simulink model "simulation_composite"  (Simulink 6.6)
settings: Solver=ode45  StartTime=0.0  StopTime=10.0  RelTol=1e-3
values from neighbouring files (symbols this model uses):
  desired_states = [set_point.theta; set_point.omega]    [set_parameters.m]    (also in tablesat3.m = str2num(get(handles.set_points,'String')))
  measurement_noise = evalin('base','measurement_noise')    [tablesat3.m]
  PID = evalin('base','PID')    [tablesat3.m]
  process_noise = evalin('base','process_noise')    [tablesat3.m]
undefined symbols (not defined in the file or in its folder): flag, plant
settings Model: Creator=Cooch  LastModifiedBy=Administrator
settings DebuggingCC: AlgebraicLoopMsg=none  SolverPrmCheckMsg=none  UnconnectedInputMsg=none  UnconnectedOutputMsg=none  UnconnectedLineMsg=none

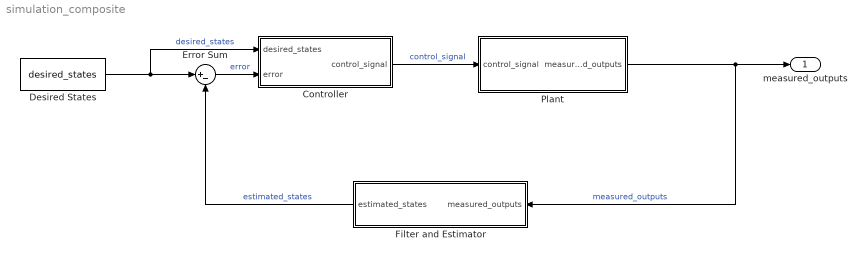
== system simulation_composite ==
  Controller : Subsystem
  Desired States : Constant  Value=desired_states
  Error Sum : Sum  Inputs=|+-
  Filter and Estimator : Subsystem  Orientation=left
  Plant : Subsystem
  measured_outputs : Outport
  wires:
  Desired States/1 -> Error Sum/1, Controller/1(desired_states)  "desired_states"
  Error Sum/1 -> Controller/2(error)  "error"
  Controller/1(control_signal) -> Plant/1(control_signal)  "control_signal"
  Filter and Estimator/1(estimated_states) -> Error Sum/2  "estimated_states"
  Plant/1(measured_outputs) -> Filter and Estimator/1(measured_outputs), measured_outputs/1  "measured_outputs"

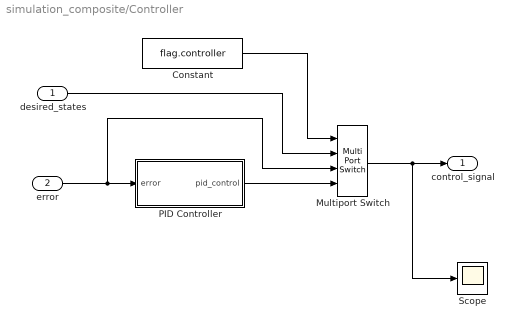
== system simulation_composite/Controller ==
  desired_states : Inport
  error : Inport  Port=2
  Constant : Constant  Value=flag.controller
  Multiport Switch : MultiPortSwitch  Inputs=3  zeroidx=on
  PID Controller : Subsystem
  Scope : Scope
  control_signal : Outport
  wires:
  error/1 -> PID Controller/1(error), Multiport Switch/3
  Multiport Switch/1 -> control_signal/1, Scope/1
  Constant/1 -> Multiport Switch/1
  PID Controller/1(pid_control) -> Multiport Switch/4
  desired_states/1 -> Multiport Switch/2

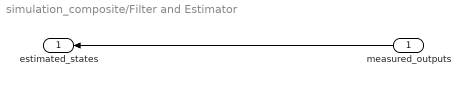
== system simulation_composite/Filter and Estimator ==
  measured_outputs : Inport  Orientation=left
  estimated_states : Outport  Orientation=left
  wires:
  measured_outputs/1 -> estimated_states/1

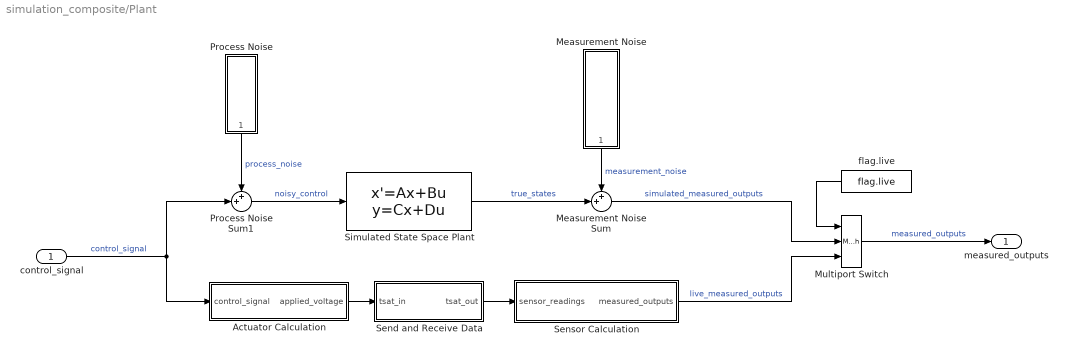
== system simulation_composite/Plant ==
  control_signal : Inport
  Actuator Calculation : Subsystem
  Measurement Noise : Subsystem  Orientation=down
  Measurement Noise Sum : Sum  Inputs=++|
  Multiport Switch : MultiPortSwitch  Inputs=2  zeroidx=on
  Process Noise : Subsystem  Orientation=down
  Process Noise Sum1 : Sum  Inputs=++|
  Send and Receive Data : Subsystem
  Sensor Calculation : Subsystem
  Simulated State Space Plant : StateSpace  A=plant.A  B=plant.B  C=plant.C  D=plant.D  X0=plant.ic
  flag.live : Constant  Orientation=left  Value=flag.live
  measured_outputs : Outport
  wires:
  Actuator Calculation/1(applied_voltage) -> Send and Receive Data/1(tsat_in)
  Send and Receive Data/1(tsat_out) -> Sensor Calculation/1(sensor_readings)
  Measurement Noise/1(measurement_noise) -> Measurement Noise Sum/1  "measurement_noise"
  Simulated State Space Plant/1 -> Measurement Noise Sum/2  "true_states"
  Multiport Switch/1 -> measured_outputs/1  "measured_outputs"
  flag.live/1 -> Multiport Switch/1
  Measurement Noise Sum/1 -> Multiport Switch/2  "simulated_measured_outputs"
  Sensor Calculation/1(measured_outputs) -> Multiport Switch/3  "live_measured_outputs"
  Process Noise/1(process_noise) -> Process Noise Sum1/1  "process_noise"
  Process Noise Sum1/1 -> Simulated State Space Plant/1  "noisy_control"
  control_signal/1 -> Process Noise Sum1/2, Actuator Calculation/1(control_signal)  "control_signal"

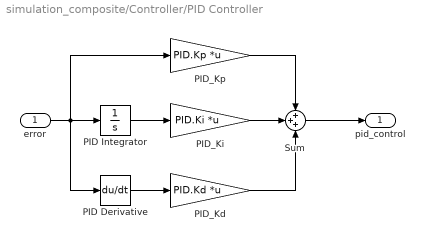
== system simulation_composite/Controller/PID Controller ==
  error : Inport
  PID Derivative : Derivative
  PID Integrator : Integrator
  PID_Kd : Gain  Gain=PID.Kd  Multiplication=Matrix(K*u)
  PID_Ki : Gain  Gain=PID.Ki  Multiplication=Matrix(K*u)
  PID_Kp : Gain  Gain=PID.Kp  Multiplication=Matrix(K*u)
  Sum : Sum  Inputs=+++
  pid_control : Outport
  wires:
  PID Integrator/1 -> PID_Ki/1
  PID Derivative/1 -> PID_Kd/1
  PID_Kp/1 -> Sum/1
  error/1 -> PID_Kp/1, PID Integrator/1, PID Derivative/1
  PID_Ki/1 -> Sum/2
  PID_Kd/1 -> Sum/3
  Sum/1 -> pid_control/1

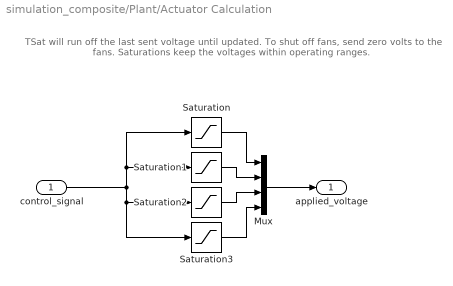
== system simulation_composite/Plant/Actuator Calculation ==
  note: TSat will run off the last sent voltage until updated.
      | To shut off fans, send zero volts to the fans.
      |
      | Saturations keep the voltages within operating ranges.
  control_signal : Inport
  Mux : Mux
  Saturation{,1..3} (4 alike) : Saturate  UpperLimit=12  LowerLimit=0
  applied_voltage : Outport
  wires:
  control_signal/1 -> Saturation/1, Saturation1/1, Saturation2/1, Saturation3/1
  Saturation/1 -> Mux/1
  Saturation1/1 -> Mux/2
  Saturation2/1 -> Mux/3
  Saturation3/1 -> Mux/4
  Mux/1 -> applied_voltage/1

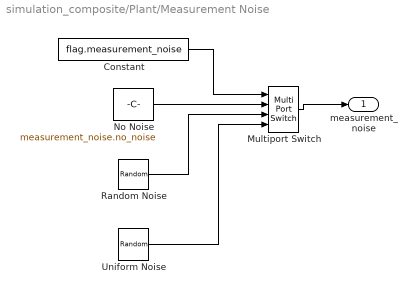
== system simulation_composite/Plant/Measurement Noise ==
  Constant : Constant  Value=flag.measurement_noise
  Multiport Switch : MultiPortSwitch  Inputs=3  zeroidx=on
  No Noise : Constant  Value=measurement_noise.no_noise
  Random Noise : RandomNumber  Mean=measurement_noise.random.mean  Variance=measurement_noise.random.variance  SampleTime=0
  Uniform Noise : UniformRandomNumber  Minimum=measurement_noise.uniform.min  Maximum=measurement_noise.uniform.max  SampleTime=0
  measurement_noise : Outport
  wires:
  Uniform Noise/1 -> Multiport Switch/4
  Constant/1 -> Multiport Switch/1
  No Noise/1 -> Multiport Switch/2
  Random Noise/1 -> Multiport Switch/3
  Multiport Switch/1 -> measurement_noise/1

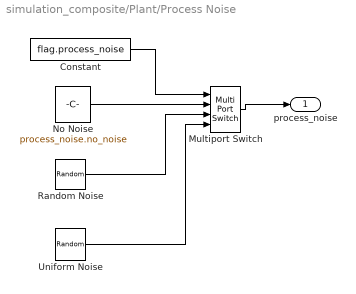
== system simulation_composite/Plant/Process Noise ==
  Constant : Constant  Value=flag.process_noise
  Multiport Switch : MultiPortSwitch  Inputs=3  zeroidx=on
  No Noise : Constant  Value=process_noise.no_noise
  Random Noise : RandomNumber  Mean=process_noise.random.mean  Variance=process_noise.random.variance  SampleTime=0
  Uniform Noise : UniformRandomNumber  Minimum=process_noise.uniform.min  Maximum=process_noise.uniform.max  SampleTime=0
  process_noise : Outport
  wires:
  Constant/1 -> Multiport Switch/1
  No Noise/1 -> Multiport Switch/2
  Random Noise/1 -> Multiport Switch/3
  Multiport Switch/1 -> process_noise/1
  Uniform Noise/1 -> Multiport Switch/4

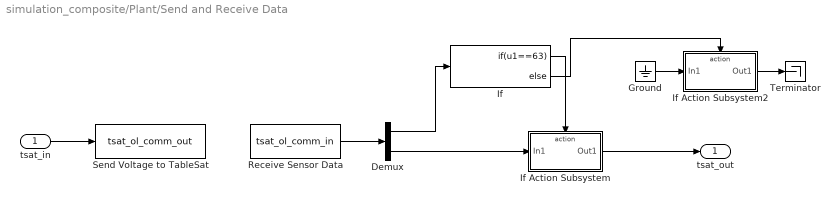
== system simulation_composite/Plant/Send and Receive Data ==
  tsat_in : Inport
  Demux : Demux  Outputs=[1;-1]
  Ground : Ground
  If : If  IfExpression=u1==63
  If Action Subsystem : Subsystem  TreatAsAtomicUnit=on
  If Action Subsystem2 : Subsystem  TreatAsAtomicUnit=on
  Receive Sensor Data : S-Function  FunctionName=tsat_ol_comm_in
  Send Voltage to TableSat : S-Function  FunctionName=tsat_ol_comm_out
  Terminator : Terminator
  tsat_out : Outport
  wires:
  tsat_in/1 -> Send Voltage to TableSat/1
  If/1 -> If Action Subsystem/Action
  If/2 -> If Action Subsystem2/Action
  Demux/1 -> If/1
  Receive Sensor Data/1 -> Demux/1
  If Action Subsystem2/1(Out1) -> Terminator/1
  Demux/2 -> If Action Subsystem/1(In1)
  Ground/1 -> If Action Subsystem2/1(In1)
  If Action Subsystem/1(Out1) -> tsat_out/1

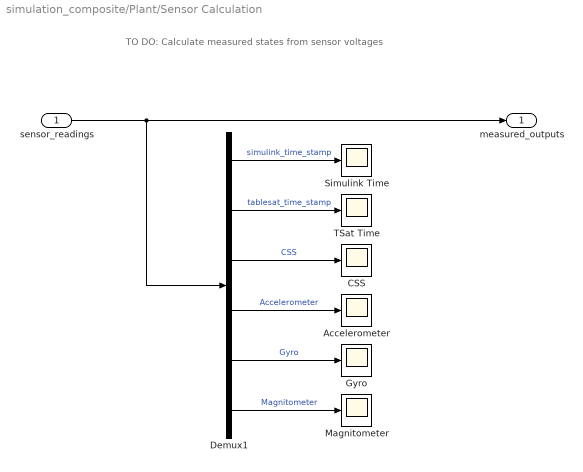
== system simulation_composite/Plant/Sensor Calculation ==
  note: TO DO: Calculate measured states from sensor voltages
  sensor_readings : Inport
  Accelerometer : Scope
      settings: YMin=2.5  YMax=4.25  SaveName=ScopeData4
  CSS : Scope
      settings: SaveName=ScopeData3
  Demux1 : Demux  Outputs=[1;1;6;4;1;3]
  Gyro : Scope
      settings: SaveName=ScopeData5
  Magnitometer : Scope
      settings: SaveName=ScopeData6
  Simulink Time : Scope
      settings: TimeRange=10  YMin=0  YMax=10
  TSat Time : Scope
      settings: SaveName=ScopeData2
  measured_outputs : Outport
  wires:
  Demux1/1 -> Simulink Time/1  "simulink_time_stamp"
  Demux1/2 -> TSat Time/1  "tablesat_time_stamp"
  Demux1/3 -> CSS/1  "CSS"
  Demux1/4 -> Accelerometer/1  "Accelerometer"
  Demux1/5 -> Gyro/1  "Gyro"
  Demux1/6 -> Magnitometer/1  "Magnitometer"
  sensor_readings/1 -> Demux1/1, measured_outputs/1

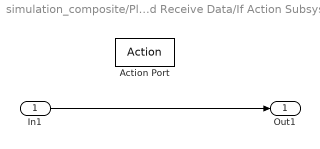
== system simulation_composite/Plant/Send and Receive Data/If Action Subsystem ==
  In1 : Inport
  Action Port : ActionPort
  Out1 : Outport
  wires:
  In1/1 -> Out1/1

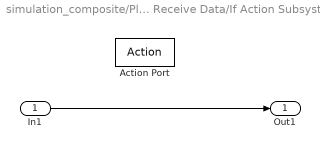
== system simulation_composite/Plant/Send and Receive Data/If Action Subsystem2 ==
  In1 : Inport
  Action Port : ActionPort
  Out1 : Outport
  wires:
  In1/1 -> Out1/1
